simulink model "chart_matlab"  (R2016a)
settings: Solver=FixedStepDiscrete  StartTime=0.0  StopTime=10.0  RelTol=1e-3
settings Model: Creator=LEGION  LastModifiedBy=LEGION
settings OptimizationCC: DefaultParameterBehavior=Inlined  OptimizeModelRefInitCode=on  LifeSpan=1
settings RTWCC: SystemTargetFile=ert.tlc  GenCodeOnly=on  TemplateMakefile=ert_default_tmf  GenerateReport=on  IncludeHyperlinkInReport=on  LaunchReport=on  GenerateTraceInfo=on  GenerateTraceReport=on  GenerateTraceReportSl=on  GenerateTraceReportSf=on  GenerateTraceReportEml=on
settings CodeAppCC: ForceParamTrailComments=on  IgnoreCustomStorageClasses=off  OperatorAnnotations=on  SimulinkDataObjDesc=on  SFDataObjDesc=on  MATLABFcnDesc=on  InsertBlockDesc=on  MATLABSourceComments=on
settings ERTTargetCC: GenerateSampleERTMain=on  InlinedParameterPlacement=NonHierarchical  ERTCustomFileTemplate=example_file_process.tlc

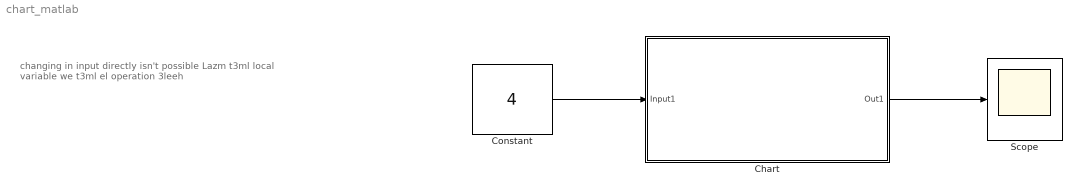
== system chart_matlab ==
  note: changing in input directly isn't possible
      |
      | Lazm t3ml local variable we t3ml el operation 3leeh
  Chart : Stateflow chart  TreatAsAtomicUnit=on
  Constant : Constant  Value=4  OutDataTypeStr=uint8
  Scope : Scope
  wires:
  Chart/1(Out1) -> Scope/1
  Constant/1 -> Chart/1(Input1)

== stateflow chart chart_matlab/Chart ==
  note: state is like the c's switch case
  note: Do not put any code along
      | the transitions that run
      | down the right side!
  note: Ay 7aga ma been [ ] 2smha transition condition;
      |
      | if the condition is valid it goes to the transition action
  (default) -> (junction 14) [order 1] : % Trial
  (junction 14) -> (junction 15) [order 1] : [Input1==1]
  (junction 14) -> (junction 16) [order 2] : {Out1=1;}
  (junction 15) -> (junction 17) : {Out1=1;}
  (junction 17) -> (junction 16)
  (default) -> (junction 27) [order 2] : /* //for loop */
  (junction 16) -> (junction 18)
  (junction 28) -> (junction 26) [order 1] : [i<10]
  (junction 26) -> (junction 29) : {printf("I am bored af");}
  (junction 27) -> (junction 28) : {i=0;}
  (junction 29) -> (junction 28) : {i++;}
  (junction 28) -> ?
  (junction 28) -> (junction 57) [order 2] : /* //switch case trials */
  (junction 57) -> (junction 58) [order 1] : [i==8]
  (junction 57) -> (junction 61) [order 2]
  (junction 58) -> (junction 59) : {i=8;}
  (junction 59) -> (junction 60)
  (junction 60) -> (junction 64)
  (junction 61) -> (junction 62) [order 1] : [i==3]
  (junction 61) -> (junction 65) [order 2]
  (junction 62) -> (junction 63) : {i=3;}
  (junction 63) -> (junction 64)
  (junction 64) -> (junction 68)
  (junction 65) -> (junction 66) [order 1] : [i==7]
  (junction 65) -> (junction 69) [order 2]
  (junction 66) -> (junction 67) : {i=1;}
  (junction 67) -> (junction 68)
  (junction 68) -> (junction 72)
  (junction 69) -> (junction 70) [order 1] : [i==9]
  (junction 69) -> (junction 73) [order 2] : {i=6;}
  (junction 70) -> (junction 71) : {i=2;}
  (junction 71) -> (junction 72)
  (junction 72) -> (junction 74)
  (junction 74) -> (junction 73)
  (junction 73) -> (junction 75)
  data: Input1 input uint8 =0; Out1 output; data local double; i local uint8
